simulink model "sampleModel18"  (R2021b)
settings: Solver=VariableStepAuto  StartTime=0.0  StopTime=10.0  RelTol=1e-3
undefined symbols (not defined in the file or in its folder): DiscIntNeverNeededParam, Newton, Raphson
libraries: simulink x15
settings Model: Creator=user  LastModifiedBy=user

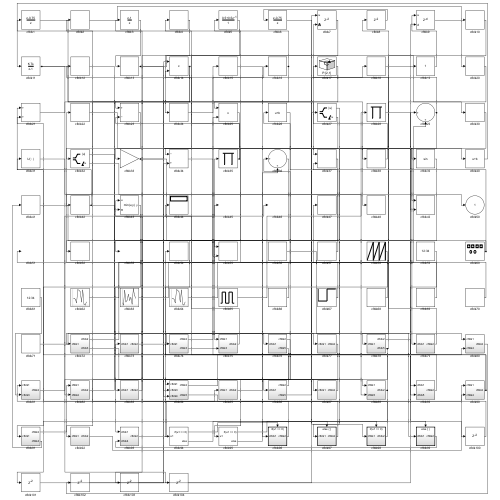
[thumbnail: Simulink's stored preview of the top-level diagram]
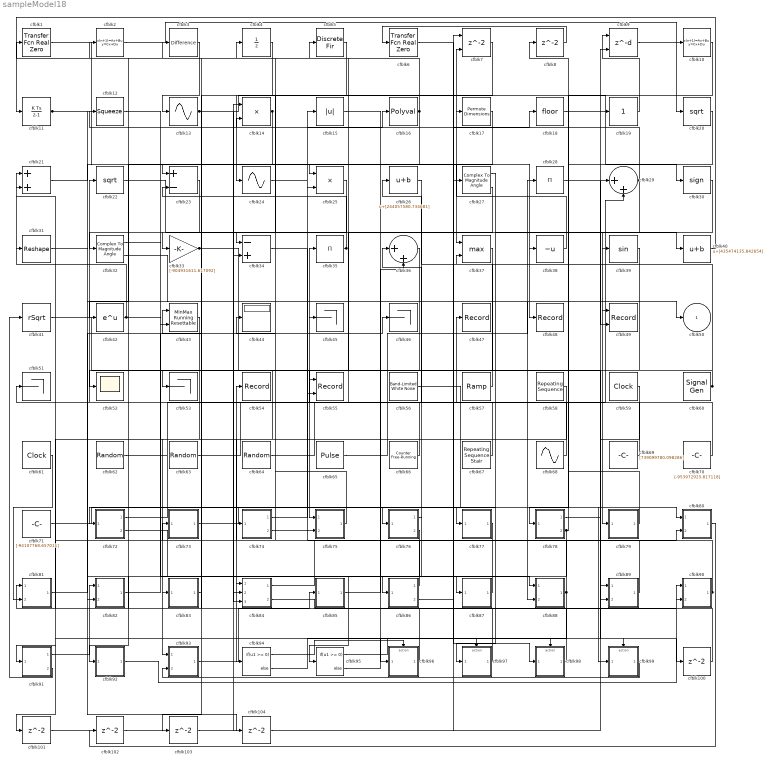
== system sampleModel18 ==
  cfblk1 : simulink/Discrete/Transfer Fcn Real Zero  ZeroZ=0.75  ICPrevInput=0.0  DoSatur=off
      settings: SourceProductBaseCode=SL
  cfblk10 : DiscreteStateSpace
  cfblk{8,100..104} (6 alike) : Delay  SampleTime=1
  cfblk11 : DiscreteIntegrator  ICPrevOutput=DiscIntNeverNeededParam  ICPrevScaledInput=DiscIntNeverNeededParam
  cfblk12 : Squeeze
  cfblk13 : Sin  TimeSource=Use external signal  SampleTime=0
  cfblk14 : Product
  cfblk15 : Abs
  cfblk16 : Polyval  Coefs=[ +2.081618890e-019, -1.441693666e-014, +4.719686976e-010, -8.536869453e-006, +1.621573104e-001, -8.087801117e+001 ]
  cfblk17 : PermuteDimensions
  cfblk18 : Rounding
  cfblk19 : simulink/Math Operations/Slider Gain  gain=1  low=0  high=2
  cfblk2 : DiscreteStateSpace
  cfblk20 : Sqrt  SaturateOnIntegerOverflow=on
  cfblk21 : Sum
  cfblk22 : Sqrt  SaturateOnIntegerOverflow=on
  cfblk23 : Sum  Inputs=+-
  cfblk24 : Sin  TimeSource=Use external signal  SampleTime=0
  cfblk25 : Product  Inputs=**
  cfblk26 : Bias  Bias=[244057580.734681]
  cfblk27 : ComplexToMagnitudeAngle
  cfblk28 : Product  Inputs=*
  cfblk29 : Sum  Inputs=|++
  cfblk3 : simulink/Discrete/Difference  ICPrevInput=0.0  OutMin=[]  OutMax=[]  OutDataTypeStr=Inherit: Inherit via back propagation  OutDataType=fixdt(1, 16)  OutScaling=2^-10  DoSatur=off
  cfblk30 : Signum
  cfblk31 : Reshape
  cfblk32 : ComplexToMagnitudeAngle
  cfblk33 : Gain  Gain=[-904931611.617092]
  cfblk34 : Sum  Inputs=-+
  cfblk35 : Product  Inputs=*
  cfblk36 : Sum  Inputs=|++
  cfblk37 : MinMax  Function=max  Inputs=2
  cfblk38 : UnaryMinus
  cfblk39 : Trigonometry
  cfblk4 : UnitDelay  HasFrameUpgradeWarning=on
  cfblk40 : Bias  Bias=[435474135.842654]
  cfblk41 : Sqrt  Operator=rSqrt  AlgorithmType=Newton-Raphson  SaturateOnIntegerOverflow=on
  cfblk42 : Math  SaturateOnIntegerOverflow=on
  cfblk43 : simulink/Math Operations/MinMax Running Resettable  Function=min  vinit=0.0
  cfblk44 : Display
  cfblk{45..46,51,53} (4 alike) : Terminator
  cfblk47 : Record  FileSettingsInternal="{\"entries\":[{\"content\":{\"excelSettings\":{\"content\":{},\"type\":\"Streamout.ExcelSettings\"}},\"type\":\"Streamout.FileSettingStorage\",\"uuid\":\"f3e6356d-f438-4730-ad7d-e3ec913a7e49\"}],\"packageUris\":[\"http://schema.mathworks.com/mf0/streamout_blocks/R2020a\"],\"version\":\"1.0\"}"  SignalsInternal="{\"entries\":[{\"content\":{\"signals\":[{\"content\":{\"blockPath\":[\"sampleModel18/cfblk47\"],\"channel\":[],\"dimensions\":[1],\"domain\":\"sampleModel18/cfblk47\",\"lineColor\":\"#a2142f\",\"plots\":[1],\"port\":1,\"sid\":[\"\"],\"signalID\":754,\"signalName\":\"cfblk67\"},\"type\":\"RecordBlkView.Signal\",\"uuid\":\"009bd073-cccd-4c9b-abca-75d434df984e\"}]},\"type\":\"RecordBlkView.InputSignals\",\"uuid\":\"1139e3b9-48b1-4a59-a758-ea53e15d3541\"}],\"packageUris\":[\"http://schema.mathworks.com/mf0/streamout_blocks/R2020a\"],\"version\":\"1.0\"}"  VisualizationBindings="{\"sparklinesplugin\":{\"info\":[{\"bindingParametersList\":[],\"subplotID\":1}]}}"
  cfblk48 : Record  FileSettingsInternal="{\"entries\":[{\"content\":{\"excelSettings\":{\"content\":{},\"type\":\"Streamout.ExcelSettings\"}},\"type\":\"Streamout.FileSettingStorage\",\"uuid\":\"b3cbeff4-dd58-4c58-a9d8-50ed42b7b65e\"}],\"packageUris\":[\"http://schema.mathworks.com/mf0/streamout_blocks/R2020a\"],\"version\":\"1.0\"}"  SignalsInternal="{\"entries\":[{\"content\":{\"signals\":[{\"content\":{\"blockPath\":[\"sampleModel18/cfblk48\"],\"channel\":[],\"dimensions\":[1],\"domain\":\"sampleModel18/cfblk48\",\"lineColor\":\"#0072bd\",\"plots\":[1],\"port\":1,\"sid\":[\"\"],\"signalID\":730,\"signalName\":\"cfblk1\"},\"type\":\"RecordBlkView.Signal\",\"uuid\":\"f6598a59-ba5a-4366-a23e-158faba5df51\"}]},\"type\":\"RecordBlkView.InputSignals\",\"uuid\":\"46017d82-f691-4fab-a069-d9b27c99119e\"}],\"packageUris\":[\"http://schema.mathworks.com/mf0/streamout_blocks/R2020a\"],\"version\":\"1.0\"}"  VisualizationBindings="{\"sparklinesplugin\":{\"info\":[{\"bindingParametersList\":[],\"subplotID\":1}]}}"
  cfblk49 : Record  FileSettingsInternal="{\"entries\":[{\"content\":{\"excelSettings\":{\"content\":{},\"type\":\"Streamout.ExcelSettings\"}},\"type\":\"Streamout.FileSettingStorage\",\"uuid\":\"12659b71-1fa3-4812-95e2-9d23bc298638\"}],\"packageUris\":[\"http://schema.mathworks.com/mf0/streamout_blocks/R2020a\"],\"version\":\"1.0\"}"  Layout=[1 1]  SignalsInternal="{\"entries\":[{\"content\":{\"signals\":[{\"content\":{\"blockPath\":[\"sampleModel18/cfblk49\"],\"channel\":[],\"dimensions\":[1],\"domain\":\"sampleModel18/cfblk49\",\"lineColor\":\"#a2142f\",\"plots\":[1],\"port\":1,\"sid\":[\"\"],\"signalID\":734,\"signalName\":\"cfblk30\"},\"type\":\"RecordBlkView.Signal\",\"uuid\":\"b456594d-3354-477f-bd82-e2a85ebed91f\"},{\"content\":{\"blockPath\":[\"sampleModel18/cfblk49\"],\"channel\":[],\"dimensions\":[1],\"domain\":\"sampleModel18/cfblk49\",\"lineColor\":\"#139fff\",\"plots\":[1],\"port\":2,\"sid\":[\"\"],\"signalID\":738,\"signalName\":\"cfblk11\"},\"type\":\"RecordBlkView.Signal\",\"uuid\":\"299b86eb-0c44-4fe7-b3fa-d8c86736a96b\"}]},\"type\":\"RecordBlkView.InputSignals\",\"uuid\":\"0a3c95b3-d673-4309-8c8b-e5e60d2abe8a\"}],\"packageUris\":[\"http://schema.mathworks.com/mf0/streamout_blocks/R2020a\"],\"version\":\"1.0\"}"  VisualizationBindings="{\"xyplotplugin\":{\"info\":[{\"series\":[{\"bindingParametersList\":[{\"parameter\":\"X-Axis\",\"signalID\":734,\"signalName\":\"cfblk30\"},{\"parameter\":\"Y-Axis\",\"signalID\":738,\"signalName\":\"cfblk11\"}],\"seriesID\":48500}],\"subplotID\":1}]}}"  CompatibilityTag=XY
  cfblk5 : DiscreteFir  SampleTime=1
  cfblk52 : Scope
  cfblk54 : Record  FileSettingsInternal="{\"entries\":[{\"content\":{\"excelSettings\":{\"content\":{},\"type\":\"Streamout.ExcelSettings\"}},\"type\":\"Streamout.FileSettingStorage\",\"uuid\":\"8c2c62a5-b023-49fb-ade8-a6f0d940a0a6\"}],\"packageUris\":[\"http://schema.mathworks.com/mf0/streamout_blocks/R2020a\"],\"version\":\"1.0\"}"  SignalsInternal="{\"entries\":[{\"content\":{\"signals\":[{\"content\":{\"blockPath\":[\"sampleModel18/cfblk54\"],\"channel\":[],\"dimensions\":[1],\"domain\":\"sampleModel18/cfblk54\",\"lineColor\":\"#7e2f8e\",\"plots\":[1],\"port\":1,\"sid\":[\"\"],\"signalID\":742,\"signalName\":\"cfblk86:1\"},\"type\":\"RecordBlkView.Signal\",\"uuid\":\"cc341828-7772-4fc4-82af-9fa621df96af\"}]},\"type\":\"RecordBlkView.InputSignals\",\"uuid\":\"70a7ec1d-eb72-4259-b67c-d21e35d60033\"}],\"packageUris\":[\"http://schema.mathworks.com/mf0/streamout_blocks/R2020a\"],\"version\":\"1.0\"}"  VisualizationBindings="{\"sparklinesplugin\":{\"info\":[{\"bindingParametersList\":[],\"subplotID\":1}]}}"
  cfblk55 : Record  FileSettingsInternal="{\"entries\":[{\"content\":{\"excelSettings\":{\"content\":{},\"type\":\"Streamout.ExcelSettings\"}},\"type\":\"Streamout.FileSettingStorage\",\"uuid\":\"f3fc9ddd-07fd-4d00-b488-08ffa401512c\"}],\"packageUris\":[\"http://schema.mathworks.com/mf0/streamout_blocks/R2020a\"],\"version\":\"1.0\"}"  Layout=[1 1]  SignalsInternal="{\"entries\":[{\"content\":{\"signals\":[{\"content\":{\"blockPath\":[\"sampleModel18/cfblk55\"],\"channel\":[],\"dimensions\":[1],\"domain\":\"sampleModel18/cfblk55\",\"lineColor\":\"#a2142f\",\"plots\":[1],\"port\":1,\"sid\":[\"\"],\"signalID\":746,\"signalName\":\"cfblk27:2\"},\"type\":\"RecordBlkView.Signal\",\"uuid\":\"ca97d49d-bb3e-4e8a-9ea8-1175d8ca5de3\"},{\"content\":{\"blockPath\":[\"sampleModel18/cfblk55\"],\"channel\":[],\"dimensions\":[1,1],\"domain\":\"sampleModel18/cfblk55\",\"lineColor\":\"#139fff\",\"plots\":[1],\"port\":2,\"sid\":[\"\"],\"signalID\":750,\"signalName\":\"cfblk32:1\"},\"type\":\"RecordBlkView.Signal\",\"uuid\":\"5159f922-05a4-4578-801b-4c852eb5fb01\"}]},\"type\":\"RecordBlkView.InputSignals\",\"uuid\":\"f493d34c-1b41-42b8-b0cc-aa9e3a55eb05\"}],\"packageUris\":[\"http://schema.mathworks.com/mf0/streamout_blocks/R2020a\"],\"version\":\"1.0\"}"  VisualizationBindings="{\"xyplotplugin\":{\"info\":[{\"series\":[{\"bindingParametersList\":[{\"parameter\":\"X-Axis\",\"signalID\":746,\"signalName\":\"cfblk27:2\"},{\"parameter\":\"Y-Axis\",\"signalID\":750,\"signalName\":\"cfblk32:1\"}],\"seriesID\":32887}],\"subplotID\":1}]}}"  CompatibilityTag=XY
  cfblk56 : simulink/Sources/Band-Limited White Noise  Cov=[9270641408.781874]  Ts=0.1  seed=[877717607.000000]
  cfblk57 : simulink/Sources/Ramp  slope=[-3352.028762]  start=[26.782864]  InitialOutput=[-506715.751883]
  cfblk58 : simulink/Sources/Repeating Sequence  rep_seq_t=[0 2]  rep_seq_y=[85798913.173892, 561735701.208153]
  cfblk59 : DigitalClock
  cfblk6 : simulink/Discrete/Transfer Fcn Real Zero  ZeroZ=0.75  ICPrevInput=0.0  DoSatur=off
      settings: SourceProductBaseCode=SL
  cfblk60 : SignalGenerator  WaveForm=sawtooth  Amplitude=[43764762.818563]  Units=rad/sec
  cfblk61 : DigitalClock
  cfblk62 : RandomNumber  Mean=[-16646.859650]  Variance=[28029.286662]  Seed=[598100317.000000]  SampleTime=0.1
  cfblk63 : UniformRandomNumber  Minimum=[-9635251432.988684]  Maximum=[636865030.513627]  Seed=[32288251.000000]  SampleTime=0.1
  cfblk64 : RandomNumber  Mean=[-80324.293923]  Variance=[17004.462627]  Seed=[371163799.000000]  SampleTime=0.1
  cfblk65 : DiscretePulseGenerator  PulseType=Time based  Amplitude=[-920476754.757523]  Period=[70924095.644116]  PulseWidth=5  PhaseDelay=[6.000000]
  cfblk66 : simulink/Sources/Counter Free-Running  NumBits=[11.000000]  tsamp=-1
  cfblk67 : simulink/Sources/Repeating Sequence Stair  OutValues=[-875696114.732629, -186681159.404449]  tsamp=-1  OutMin=[]  OutMax=[]  OutDataTypeStr=double  OutputDataTypeScalingMode=double  OutDataType=fixdt(0,8)  ConRadixGroup=Best Precision: Vector-wise  OutScaling=2^-12
  cfblk68 : Sin  Amplitude=[-73874148.181670]  Bias=[-594651401.125389]  SampleTime=0
  cfblk69 : Constant  Value=[739099780.098286]  SampleTime=1
  cfblk7 : Delay  ShowEnablePort=on  SampleTime=1
      settings: InputPortMap=u0,e6
  cfblk70 : Constant  Value=[-953972925.817118]  SampleTime=1
  cfblk71 : Constant  Value=[-94107768.657011]  SampleTime=1
  cfblk72 : Subsystem
  cfblk73 : Subsystem
  cfblk74 : Subsystem
  cfblk75 : Subsystem
  cfblk76 : Subsystem
  cfblk77 : Subsystem
  cfblk78 : Subsystem
  cfblk79 : Subsystem
  cfblk80 : Subsystem
  cfblk81 : Subsystem
  cfblk82 : Subsystem
  cfblk83 : Subsystem
  cfblk84 : Subsystem
  cfblk85 : Subsystem
  cfblk86 : Subsystem
  cfblk87 : Subsystem
  cfblk88 : Subsystem
  cfblk89 : Subsystem
  cfblk9 : Delay  DelayLengthSource=Input port  SampleTime=1
      settings: InputPortMap=u0,p1
  cfblk90 : Subsystem
  cfblk91 : Subsystem
  cfblk92 : Subsystem
  cfblk93 : Subsystem
  cfblk94 : If  IfExpression=u1 >= 0  SampleTime=1
  cfblk95 : If  IfExpression=u1 >= 0  SampleTime=1
  cfblk96 : Subsystem  TreatAsAtomicUnit=on
  cfblk97 : Subsystem  TreatAsAtomicUnit=on
  cfblk98 : Subsystem  TreatAsAtomicUnit=on
  cfblk99 : Subsystem  TreatAsAtomicUnit=on
  cfblk50 : Outport
  wires:
  cfblk8/1 -> cfblk6/1
  cfblk36/1 -> cfblk53/1
  cfblk86/1(cfblk2) -> cfblk54/1
  cfblk98/1(cfblk2) -> cfblk81/1(cfblk1)
  cfblk91/1(cfblk2) -> cfblk82/1(cfblk1)
  cfblk22/1 -> cfblk79/1(cfblk1)
  cfblk71/1 -> cfblk76/1(cfblk1)
  cfblk76/1(cfblk2) -> cfblk82/2(cfblk4)
  cfblk57/1 -> cfblk26/1
  cfblk61/1 -> cfblk81/2(cfblk3)
  cfblk15/1 -> cfblk96/1(cfblk1)
  cfblk77/1(cfblk2) -> cfblk92/1(cfblk1)
  cfblk66/1 -> cfblk22/1
  cfblk11/1 -> cfblk37/1, cfblk49/2
  cfblk96/1(cfblk2) -> cfblk43/1
  cfblk63/1 -> cfblk35/1
  cfblk19/1 -> cfblk9/1
  cfblk3/1 -> cfblk13/1
  cfblk21/1 -> cfblk23/1
  cfblk13/1 -> cfblk30/1, cfblk39/1
  cfblk56/1 -> cfblk99/1(cfblk1)
  cfblk25/1 -> cfblk32/1
  cfblk43/1 -> cfblk93/1(cfblk1)
  cfblk1/1 -> cfblk48/1
  cfblk81/1(cfblk2) -> cfblk46/1
  cfblk60/1 -> cfblk52/1, cfblk37/2
  cfblk93/1(cfblk2) -> cfblk85/1(cfblk1)
  cfblk83/1(cfblk2) -> cfblk23/2
  cfblk2/1 -> cfblk20/1
  cfblk5/1 -> cfblk24/1
  cfblk40/1 -> cfblk11/1
  cfblk73/1(cfblk2) -> cfblk80/1(cfblk1)
  cfblk41/1 -> cfblk75/1(cfblk1)
  cfblk99/1(cfblk2) -> cfblk93/2(cfblk4)
  cfblk39/1 -> cfblk94/1
  cfblk33/1 -> cfblk89/1(cfblk1), cfblk40/1
  cfblk67/1 -> cfblk47/1
  cfblk26/1 -> cfblk86/1(cfblk1)
  cfblk69/1 -> cfblk51/1
  cfblk28/1 -> cfblk50/1
  cfblk17/1 -> cfblk25/1
  cfblk29/1 -> cfblk7/2, cfblk97/1(cfblk1)
  cfblk65/1 -> cfblk28/1
  cfblk6/1 -> cfblk98/1(cfblk1)
  cfblk90/1(cfblk2) -> cfblk73/1(cfblk1), cfblk31/1
  cfblk12/1 -> cfblk87/1(cfblk1)
  cfblk58/1 -> cfblk91/1(cfblk1)
  cfblk87/1(cfblk2) -> cfblk84/1(cfblk1)
  cfblk74/1(cfblk2) -> cfblk25/2
  cfblk4/1 -> cfblk83/1(cfblk1)
  cfblk35/1 -> cfblk4/1, cfblk3/1
  cfblk9/1 -> cfblk10/1
  cfblk34/1 -> cfblk75/2(cfblk3)
  cfblk20/1 -> cfblk78/1(cfblk1)
  cfblk88/1(cfblk2) -> cfblk44/1, cfblk101/1
  cfblk27/1 -> cfblk72/1(cfblk1)
  cfblk42/1 -> cfblk21/1, cfblk77/1(cfblk1)
  cfblk38/1 -> cfblk17/1
  cfblk68/1 -> cfblk5/1
  cfblk7/1 -> cfblk34/1
  cfblk14/1 -> cfblk42/1, cfblk43/2
  cfblk10/1 -> cfblk38/1
  cfblk64/1 -> cfblk19/1
  cfblk18/1 -> cfblk9/2
  cfblk70/1 -> cfblk36/1
  cfblk76/2(cfblk5) -> cfblk84/2(cfblk3)
  cfblk74/2(cfblk3) -> cfblk80/2(cfblk4)
  cfblk16/1 -> cfblk1/1, cfblk84/3(cfblk4)
  cfblk62/1 -> cfblk15/1
  cfblk27/2 -> cfblk55/1
  cfblk84/1(cfblk2) -> cfblk27/1
  cfblk72/1(cfblk2) -> cfblk29/2
  cfblk75/1(cfblk2) -> cfblk14/2
  cfblk92/1(cfblk2) -> cfblk90/1(cfblk1)
  cfblk85/1(cfblk2) -> cfblk36/2
  cfblk97/1(cfblk2) -> cfblk21/2
  cfblk30/1 -> cfblk49/1
  cfblk79/1(cfblk2) -> cfblk8/1
  cfblk23/1 -> cfblk33/1
  cfblk24/1 -> cfblk16/1
  cfblk89/1(cfblk2) -> cfblk74/1(cfblk1)
  cfblk72/2(cfblk3) -> cfblk88/1(cfblk1)
  cfblk84/2(cfblk5) -> cfblk90/2(cfblk4)
  cfblk82/1(cfblk2) -> cfblk45/1
  cfblk91/2(cfblk4) -> cfblk41/1
  cfblk86/2(cfblk5) -> cfblk18/1
  cfblk59/1 -> cfblk89/2(cfblk5)
  cfblk32/1 -> cfblk55/2
  cfblk78/2(cfblk5) -> cfblk12/1, cfblk95/1
  cfblk32/2 -> cfblk88/2(cfblk5)
  cfblk94/1 -> cfblk96/Action
  cfblk94/2 -> cfblk97/Action
  cfblk95/1 -> cfblk98/Action
  cfblk95/2 -> cfblk99/Action
  cfblk78/1(cfblk2) -> cfblk100/1
  cfblk100/1 -> cfblk2/1
  cfblk101/1 -> cfblk34/2
  cfblk80/1(cfblk2) -> cfblk102/1
  cfblk102/1 -> cfblk14/1
  cfblk37/1 -> cfblk103/1
  cfblk103/1 -> cfblk29/1
  cfblk31/1 -> cfblk104/1
  cfblk104/1 -> cfblk7/1

== system sampleModel18/cfblk72 ==
  cfblk1 : Inport
  cfblk2 : Outport
  cfblk3 : Outport  Port=2
  wires:
  cfblk1/1 -> cfblk3/1, cfblk2/1

== system sampleModel18/cfblk73 ==
  cfblk1 : Inport
  cfblk3 : DiscreteFilter  SampleTime=1
  cfblk4 : PermuteDimensions
  cfblk2 : Outport
  wires:
  cfblk1/1 -> cfblk3/1
  cfblk3/1 -> cfblk2/1, cfblk4/1

== system sampleModel18/cfblk74 ==
  cfblk1 : Inport
  cfblk2 : Outport
  cfblk3 : Outport  Port=2
  wires:
  cfblk1/1 -> cfblk3/1, cfblk2/1

== system sampleModel18/cfblk75 ==
  cfblk1 : Inport
  cfblk3 : Inport  Port=2
  cfblk2 : Outport
  wires:
  cfblk1/1 -> cfblk2/1

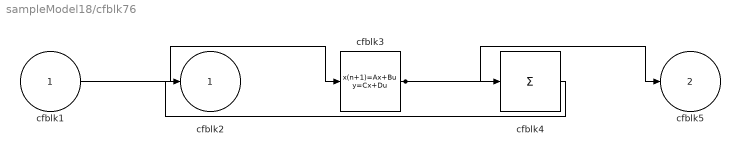
== system sampleModel18/cfblk76 ==
  cfblk1 : Inport
  cfblk3 : DiscreteStateSpace
  cfblk4 : Sum  Inputs=+
  cfblk2 : Outport
  cfblk5 : Outport  Port=2
  wires:
  cfblk1/1 -> cfblk3/1
  cfblk3/1 -> cfblk4/1, cfblk5/1
  cfblk4/1 -> cfblk2/1

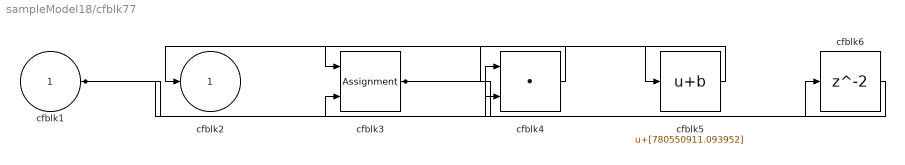
== system sampleModel18/cfblk77 ==
  cfblk1 : Inport
  cfblk3 : Assignment  DiagnosticForDimensions=Warning  IndexOptions=Index vector (dialog)  Indices=1  OutputSizes=1
  cfblk4 : DotProduct  InputSameDT=on  OutDataTypeStr=Inherit: Inherit via internal rule
  cfblk5 : Bias  Bias=[780550911.093952]
  cfblk6 : Delay  SampleTime=1
  cfblk2 : Outport
  wires:
  cfblk5/1 -> cfblk2/1
  cfblk1/1 -> cfblk4/1, cfblk3/2
  cfblk3/1 -> cfblk5/1, cfblk6/1
  cfblk4/1 -> cfblk3/1
  cfblk6/1 -> cfblk4/2

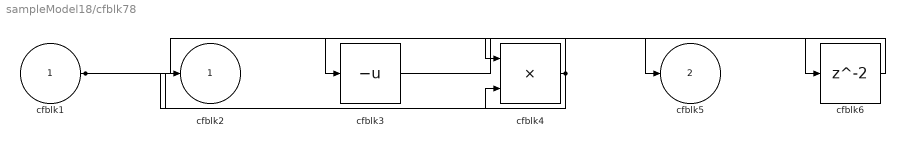
== system sampleModel18/cfblk78 ==
  cfblk1 : Inport
  cfblk3 : UnaryMinus
  cfblk4 : Product
  cfblk6 : Delay  SampleTime=1
  cfblk2 : Outport
  cfblk5 : Outport  Port=2
  wires:
  cfblk1/1 -> cfblk5/1, cfblk4/2
  cfblk4/1 -> cfblk2/1, cfblk3/1
  cfblk3/1 -> cfblk6/1
  cfblk6/1 -> cfblk4/1

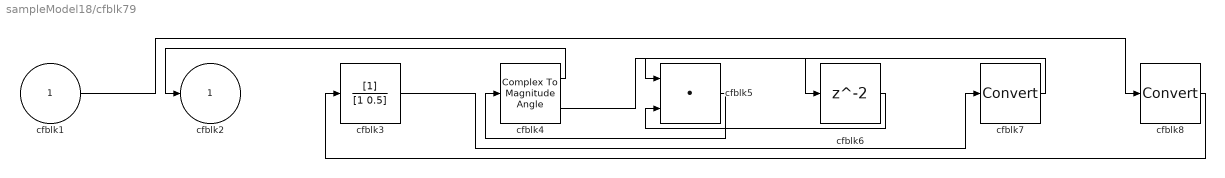
== system sampleModel18/cfblk79 ==
  cfblk1 : Inport
  cfblk3 : DiscreteFilter  SampleTime=1
  cfblk4 : ComplexToMagnitudeAngle
  cfblk5 : DotProduct  InputSameDT=on  OutDataTypeStr=Inherit: Inherit via internal rule
  cfblk6 : Delay  SampleTime=1
  cfblk7 : DataTypeConversion
  cfblk8 : DataTypeConversion
  cfblk2 : Outport
  wires:
  cfblk4/1 -> cfblk2/1
  cfblk5/1 -> cfblk4/1
  cfblk4/2 -> cfblk6/1
  cfblk6/1 -> cfblk5/2
  cfblk3/1 -> cfblk7/1
  cfblk7/1 -> cfblk5/1
  cfblk1/1 -> cfblk8/1
  cfblk8/1 -> cfblk3/1

== system sampleModel18/cfblk80 ==
  cfblk1 : Inport
  cfblk4 : Inport  Port=2
  cfblk3 : simulink/Discrete/Transfer Fcn Real Zero  ZeroZ=0.75  ICPrevInput=0.0  DoSatur=off
      settings: SourceProductBaseCode=SL
  cfblk2 : Outport
  wires:
  cfblk1/1 -> cfblk2/1
  cfblk4/1 -> cfblk3/1

== system sampleModel18/cfblk81 ==
  cfblk1 : Inport
  cfblk3 : Inport  Port=2
  cfblk2 : Outport
  wires:
  cfblk1/1 -> cfblk2/1

== system sampleModel18/cfblk82 ==
  cfblk1 : Inport
  cfblk4 : Inport  Port=2
  cfblk3 : Sum  Inputs=--
  cfblk2 : Outport
  wires:
  cfblk3/1 -> cfblk2/1
  cfblk4/1 -> cfblk3/1
  cfblk1/1 -> cfblk3/2

== system sampleModel18/cfblk83 ==
  cfblk1 : Inport
  cfblk3 : simulink/Discrete/Transfer Fcn Real Zero  ZeroZ=0.75  ICPrevInput=0.0  DoSatur=off
      settings: SourceProductBaseCode=SL
  cfblk4 : Sqrt  Operator=rSqrt  AlgorithmType=Newton-Raphson  SaturateOnIntegerOverflow=on
  cfblk2 : Outport
  wires:
  cfblk1/1 -> cfblk3/1
  cfblk3/1 -> cfblk4/1
  cfblk4/1 -> cfblk2/1

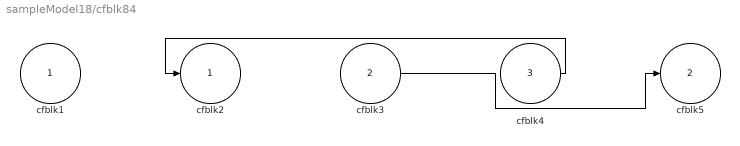
== system sampleModel18/cfblk84 ==
  cfblk1 : Inport
  cfblk3 : Inport  Port=2
  cfblk4 : Inport  Port=3
  cfblk2 : Outport
  cfblk5 : Outport  Port=2
  wires:
  cfblk4/1 -> cfblk2/1
  cfblk3/1 -> cfblk5/1

== system sampleModel18/cfblk85 ==
  cfblk1 : Inport
  cfblk3 : Delay  SampleTime=1
  cfblk4 : Constant  Value=[124001704.281891]  SampleTime=1
  cfblk2 : Outport
  wires:
  cfblk4/1 -> cfblk3/1
  cfblk3/1 -> cfblk2/1

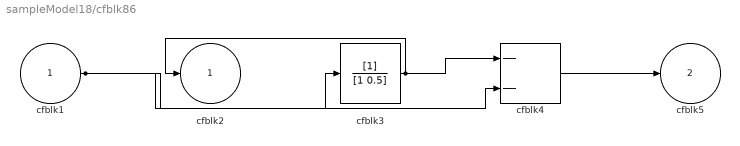
== system sampleModel18/cfblk86 ==
  cfblk1 : Inport
  cfblk3 : DiscreteFilter  SampleTime=1
  cfblk4 : Sum  Inputs=--
  cfblk2 : Outport
  cfblk5 : Outport  Port=2
  wires:
  cfblk3/1 -> cfblk2/1, cfblk4/1
  cfblk1/1 -> cfblk3/1, cfblk4/2
  cfblk4/1 -> cfblk5/1

== system sampleModel18/cfblk87 ==
  cfblk1 : Inport
  cfblk3 : Sin  TimeSource=Use external signal  SampleTime=0
  cfblk2 : Outport
  wires:
  cfblk1/1 -> cfblk3/1
  cfblk3/1 -> cfblk2/1

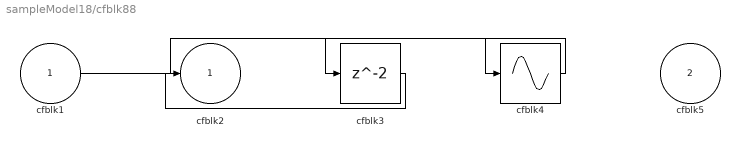
== system sampleModel18/cfblk88 ==
  cfblk1 : Inport
  cfblk5 : Inport  Port=2
  cfblk3 : Delay  SampleTime=1
  cfblk4 : Sin  TimeSource=Use external signal  SampleTime=0
  cfblk2 : Outport
  wires:
  cfblk1/1 -> cfblk4/1
  cfblk3/1 -> cfblk2/1
  cfblk4/1 -> cfblk3/1

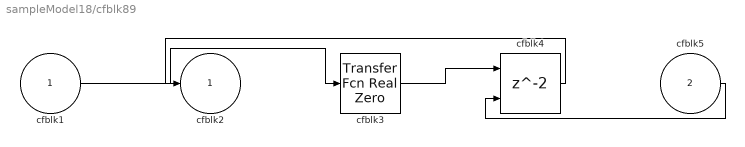
== system sampleModel18/cfblk89 ==
  cfblk1 : Inport
  cfblk5 : Inport  Port=2
  cfblk3 : simulink/Discrete/Transfer Fcn Real Zero  ZeroZ=0.75  ICPrevInput=0.0  DoSatur=off
      settings: SourceProductBaseCode=SL
  cfblk4 : Delay  ShowEnablePort=on  SampleTime=1
      settings: InputPortMap=u0,e6
  cfblk2 : Outport
  wires:
  cfblk3/1 -> cfblk4/1
  cfblk1/1 -> cfblk3/1
  cfblk5/1 -> cfblk4/2
  cfblk4/1 -> cfblk2/1

== system sampleModel18/cfblk90 ==
  cfblk1 : Inport
  cfblk4 : Inport  Port=2
  cfblk3 : Constant  Value=[370534080.999301]  SampleTime=1
  cfblk2 : Outport
  wires:
  cfblk3/1 -> cfblk2/1

== system sampleModel18/cfblk91 ==
  cfblk1 : Inport
  cfblk3 : DotProduct  InputSameDT=on  OutDataTypeStr=Inherit: Inherit via internal rule
  cfblk2 : Outport
  cfblk4 : Outport  Port=2
  wires:
  cfblk1/1 -> cfblk3/1, cfblk3/2
  cfblk3/1 -> cfblk2/1, cfblk4/1

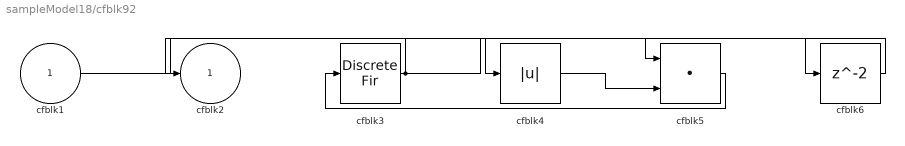
== system sampleModel18/cfblk92 ==
  cfblk1 : Inport
  cfblk3 : DiscreteFir  SampleTime=1
  cfblk4 : Abs
  cfblk5 : DotProduct  InputSameDT=on  OutDataTypeStr=Inherit: Inherit via internal rule
  cfblk6 : Delay  SampleTime=1
  cfblk2 : Outport
  wires:
  cfblk3/1 -> cfblk2/1, cfblk6/1
  cfblk1/1 -> cfblk4/1
  cfblk4/1 -> cfblk5/2
  cfblk5/1 -> cfblk3/1
  cfblk6/1 -> cfblk5/1

== system sampleModel18/cfblk93 ==
  cfblk1 : Inport
  cfblk4 : Inport  Port=2
  cfblk3 : Sqrt  SaturateOnIntegerOverflow=on
  cfblk2 : Outport
  wires:
  cfblk1/1 -> cfblk2/1
  cfblk4/1 -> cfblk3/1

== system sampleModel18/cfblk96 ==
  cfblk1 : Inport
  Action Port : ActionPort  ActionPortLabel=if(u1 >= 0)
  cfblk3 : DiscreteStateSpace  SampleTime=-1
  cfblk2 : Outport
  wires:
  cfblk1/1 -> cfblk2/1, cfblk3/1

== system sampleModel18/cfblk97 ==
  cfblk1 : Inport
  Action Port : ActionPort  ActionPortLabel=else
  cfblk3 : Sum  Inputs=+-
  cfblk4 : Constant  Value=[862950299.846338]  SampleTime=1
  cfblk2 : Outport
  wires:
  cfblk4/1 -> cfblk3/1
  cfblk1/1 -> cfblk3/2
  cfblk3/1 -> cfblk2/1

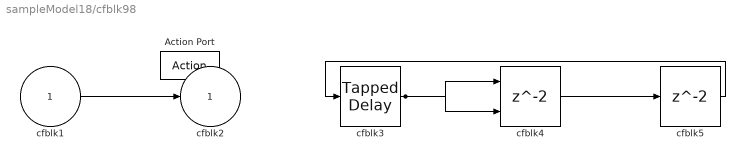
== system sampleModel18/cfblk98 ==
  cfblk1 : Inport
  Action Port : ActionPort  ActionPortLabel=if(u1 >= 0)
  cfblk3 : simulink/Discrete/Tapped Delay  vinit=0.0  samptime=-1  NumDelays=1  DelayOrder=Oldest  includeCurrent=off
  cfblk4 : Delay  ShowEnablePort=on
      settings: InputPortMap=u0,e6
  cfblk5 : Delay
  cfblk2 : Outport
  wires:
  cfblk3/1 -> cfblk4/1, cfblk4/2
  cfblk1/1 -> cfblk2/1
  cfblk4/1 -> cfblk5/1
  cfblk5/1 -> cfblk3/1

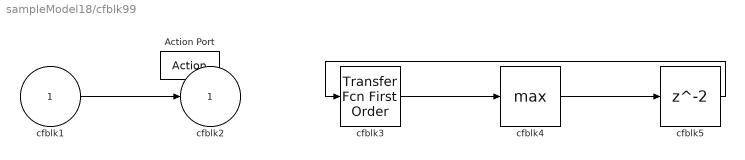
== system sampleModel18/cfblk99 ==
  cfblk1 : Inport
  Action Port : ActionPort  ActionPortLabel=else
  cfblk3 : simulink/Discrete/Transfer Fcn First Order  PoleZ=0.95  ICPrevOutput=0.0  DoSatur=off
  cfblk4 : MinMax  Function=max
  cfblk5 : Delay
  cfblk2 : Outport
  wires:
  cfblk1/1 -> cfblk2/1
  cfblk3/1 -> cfblk4/1
  cfblk4/1 -> cfblk5/1
  cfblk5/1 -> cfblk3/1
